simulink model "demo"  (R2022b)
settings: Solver=VariableStepAuto  StartTime=0.0  StopTime=1000.0  RelTol=1e-3
settings Model: Creator=mingh  LastModifiedBy=mingh

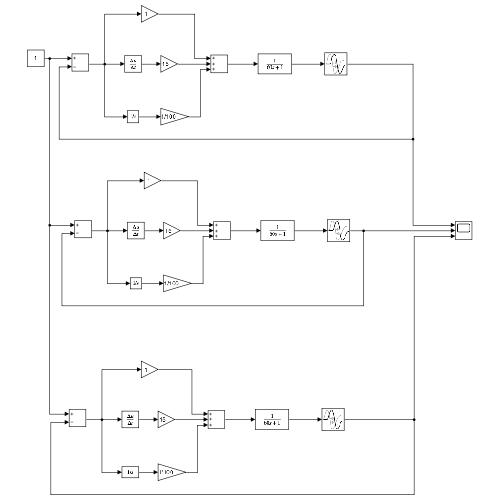
[thumbnail: Simulink's stored preview of the top-level diagram]
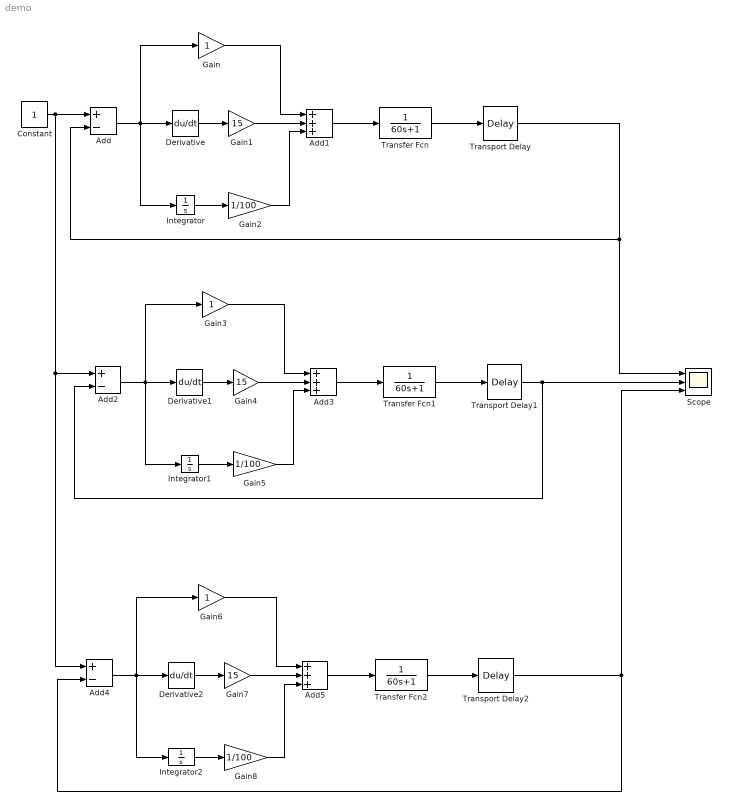
== system demo ==
  Add : Sum  Inputs=+-
  Add1 : Sum  Inputs=+++
  Add2 : Sum  Inputs=+-
  Add3 : Sum  Inputs=+++
  Add4 : Sum  Inputs=+-
  Add5 : Sum  Inputs=+++
  Constant : Constant
  Derivative : Derivative
  Derivative1 : Derivative
  Derivative2 : Derivative
  Gain : Gain
  Gain1 : Gain  Gain=15
  Gain2 : Gain  Gain=1/100
  Gain3 : Gain
  Gain4 : Gain  Gain=15
  Gain5 : Gain  Gain=1/100
  Gain6 : Gain
  Gain7 : Gain  Gain=15
  Gain8 : Gain  Gain=1/100
  Integrator : Integrator
  Integrator1 : Integrator
  Integrator2 : Integrator
  Scope : Scope  NumInputPorts=3
  Transfer Fcn : TransferFcn  Denominator=[60 1]
  Transfer Fcn1 : TransferFcn  Denominator=[60 1]
  Transfer Fcn2 : TransferFcn  Denominator=[60 1]
  Transport Delay : TransportDelay  DelayTime=80
  Transport Delay1 : TransportDelay  DelayTime=80
  Transport Delay2 : TransportDelay  DelayTime=80
  wires:
  Constant/1 -> Add4/1, Add2/1, Add/1
  Derivative/1 -> Gain1/1
  Gain/1 -> Add1/1
  Add1/1 -> Transfer Fcn/1
  Transfer Fcn/1 -> Transport Delay/1
  Transport Delay/1 -> Add/2, Scope/1
  Gain2/1 -> Add1/3
  Gain1/1 -> Add1/2
  Derivative1/1 -> Gain4/1
  Gain5/1 -> Add3/3
  Gain3/1 -> Add3/1
  Transfer Fcn1/1 -> Transport Delay1/1
  Gain4/1 -> Add3/2
  Add3/1 -> Transfer Fcn1/1
  Add2/1 -> Integrator1/1, Derivative1/1, Gain3/1
  Transport Delay1/1 -> Add2/2, Scope/2
  Integrator1/1 -> Gain5/1
  Derivative2/1 -> Gain7/1
  Gain8/1 -> Add5/3
  Gain6/1 -> Add5/1
  Transfer Fcn2/1 -> Transport Delay2/1
  Gain7/1 -> Add5/2
  Add5/1 -> Transfer Fcn2/1
  Add4/1 -> Integrator2/1, Derivative2/1, Gain6/1
  Integrator2/1 -> Gain8/1
  Transport Delay2/1 -> Scope/3, Add4/2
  Add/1 -> Gain/1, Integrator/1, Derivative/1
  Integrator/1 -> Gain2/1
